simulink model "sampleModel235"  (R2021b)
settings: Solver=VariableStepAuto  StartTime=0.0  StopTime=10.0  RelTol=1e-3
undefined symbols (not defined in the file or in its folder): Newton, Raphson
libraries: simulink x16, slpidlib x3
settings Model: Creator=user  LastModifiedBy=user

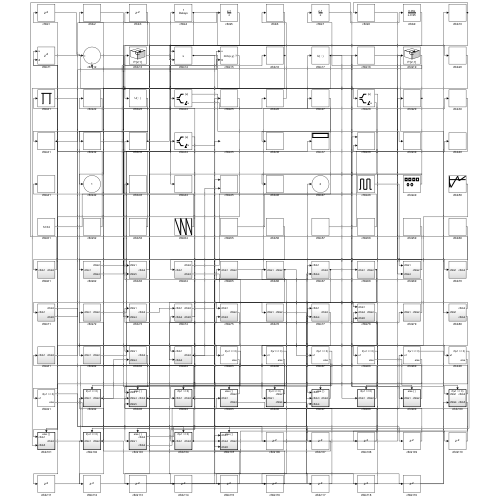
[thumbnail: Simulink's stored preview of the top-level diagram]
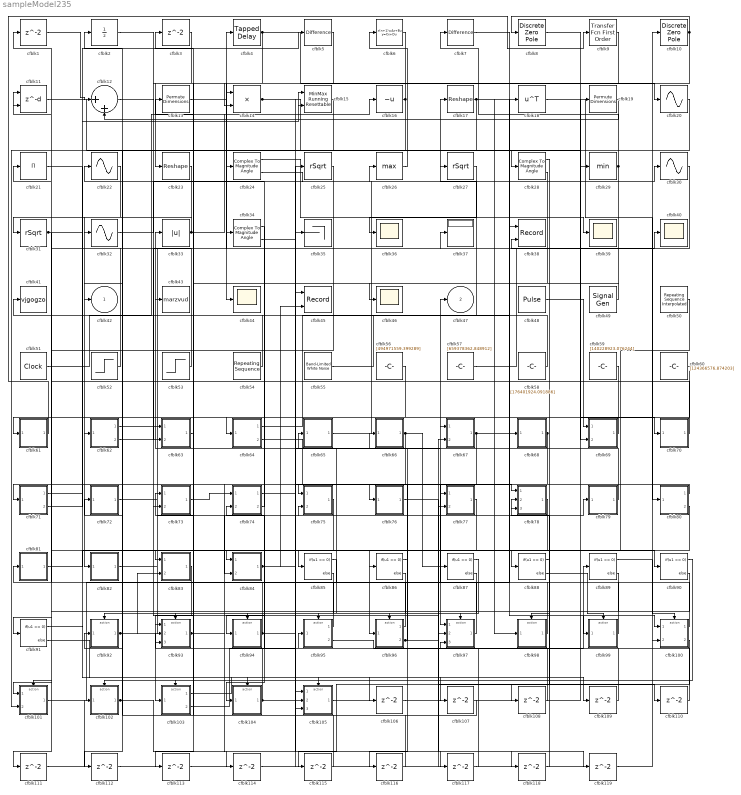
== system sampleModel235 ==
  cfblk{1,3,106..119} (16 alike) : Delay  SampleTime=1
  cfblk10 : DiscreteZeroPole  Poles=[0 0.5]  Gain=1
  cfblk100 : Subsystem  TreatAsAtomicUnit=on
  cfblk101 : Subsystem  TreatAsAtomicUnit=on
  cfblk102 : Subsystem  TreatAsAtomicUnit=on
  cfblk103 : Subsystem  TreatAsAtomicUnit=on
  cfblk104 : Subsystem  TreatAsAtomicUnit=on
  cfblk105 : Subsystem  TreatAsAtomicUnit=on
  cfblk11 : Delay  DelayLengthSource=Input port  SampleTime=1
      settings: InputPortMap=u0,p1
  cfblk12 : Sum  Inputs=|++
  cfblk13 : PermuteDimensions
  cfblk14 : Product
  cfblk15 : simulink/Math Operations/MinMax Running Resettable  Function=min  vinit=0.0
  cfblk16 : UnaryMinus
  cfblk17 : Reshape
  cfblk18 : Math  Operator=transpose  SaturateOnIntegerOverflow=on
  cfblk19 : PermuteDimensions
  cfblk2 : UnitDelay  HasFrameUpgradeWarning=on
  cfblk{20,22,30,32} (4 alike) : Sin  TimeSource=Use external signal  SampleTime=0
  cfblk21 : Product  Inputs=*
  cfblk23 : Reshape
  cfblk24 : ComplexToMagnitudeAngle
  cfblk25 : Sqrt  Operator=rSqrt  AlgorithmType=Newton-Raphson  SaturateOnIntegerOverflow=on
  cfblk26 : MinMax  Function=max
  cfblk27 : Sqrt  Operator=rSqrt  AlgorithmType=Newton-Raphson  SaturateOnIntegerOverflow=on
  cfblk28 : ComplexToMagnitudeAngle
  cfblk29 : MinMax
  cfblk31 : Sqrt  Operator=rSqrt  AlgorithmType=Newton-Raphson  SaturateOnIntegerOverflow=on
  cfblk33 : Abs
  cfblk34 : ComplexToMagnitudeAngle
  cfblk35 : Terminator
  cfblk{36,39..40,44,46} (5 alike) : Scope
  cfblk37 : Display
  cfblk38 : Record  FileSettingsInternal="{\"entries\":[{\"content\":{\"excelSettings\":{\"content\":{},\"type\":\"Streamout.ExcelSettings\"}},\"type\":\"Streamout.FileSettingStorage\",\"uuid\":\"11336398-6d51-4f3b-8d62-29296b9ae9b3\"}],\"packageUris\":[\"http://schema.mathworks.com/mf0/streamout_blocks/R2020a\"],\"version\":\"1.0\"}"  Layout=[1 1]  SignalsInternal="{\"entries\":[{\"content\":{\"signals\":[{\"content\":{\"blockPath\":[\"sampleModel235/cfblk38\"],\"channel\":[],\"dimensions\":[1],\"domain\":\"sampleModel235/cfblk38\",\"lineColor\":\"#a2142f\",\"plots\":[1],\"port\":1,\"sid\":[\"\"],\"signalID\":9263,\"signalName\":\"cfblk101\"},\"type\":\"RecordBlkView.Signal\",\"uuid\":\"63c3850a-55ea-46c7-aea2-e643b16b634b\"},{\"content\":{\"blockPath\":[\"sampleModel235/cfblk38\"],\"channel\":[],\"dimensions\":[1],\"domain\":\"sampleModel235/cfblk38\",\"lineColor\":\"#139fff\",\"plots\":[1],\"port\":2,\"sid\":[\"\"],\"signalID\":9267,\"signalName\":\"cfblk30\"},\"type\":\"RecordBlkView.Signal\",\"uuid\":\"79ddd3dd-8e78-4676-acbe-30bf93b9a830\"}]},\"type\":\"RecordBlkView.InputSignals\",\"uuid\":\"fa292d2c-9bc8-478c-a53f-73bef0c1fc4b\"}],\"packageUris\":[\"http://schema.mathworks.com/mf0/streamout_blocks/R2020a\"],\"version\":\"1.0\"}"  VisualizationBindings="{\"xyplotplugin\":{\"info\":[{\"series\":[{\"bindingParametersList\":[{\"parameter\":\"X-Axis\",\"signalID\":9263,\"signalName\":\"cfblk101\"},{\"parameter\":\"Y-Axis\",\"signalID\":9267,\"signalName\":\"cfblk30\"}],\"seriesID\":30601}],\"subplotID\":1}]}}"  CompatibilityTag=XY
  cfblk4 : simulink/Discrete/Tapped Delay  vinit=0.0  samptime=-1  NumDelays=1  DelayOrder=Oldest  includeCurrent=off
  cfblk41 : ToWorkspace  VariableName=vjgogzo  SaveFormat=Timeseries  SampleTime=-1
  cfblk43 : ToWorkspace  VariableName=marzvud  SaveFormat=Timeseries  SampleTime=-1
  cfblk45 : Record  FileSettingsInternal="{\"entries\":[{\"content\":{\"excelSettings\":{\"content\":{},\"type\":\"Streamout.ExcelSettings\"}},\"type\":\"Streamout.FileSettingStorage\",\"uuid\":\"599320f1-be0e-48c2-8f03-a9a55e95d92d\"}],\"packageUris\":[\"http://schema.mathworks.com/mf0/streamout_blocks/R2020a\"],\"version\":\"1.0\"}"  Layout=[1 1]  SignalsInternal="{\"entries\":[{\"content\":{\"signals\":[{\"content\":{\"blockPath\":[\"sampleModel235/cfblk45\"],\"channel\":[],\"dimensions\":[1],\"domain\":\"sampleModel235/cfblk45\",\"lineColor\":\"#a2142f\",\"plots\":[1],\"port\":1,\"sid\":[\"\"],\"signalID\":9271,\"signalName\":\"cfblk84\"},\"type\":\"RecordBlkView.Signal\",\"uuid\":\"f68cf5d5-64ff-4d75-8381-95ab246270b4\"},{\"content\":{\"blockPath\":[\"sampleModel235/cfblk45\"],\"channel\":[],\"dimensions\":[1],\"domain\":\"sampleModel235/cfblk45\",\"lineColor\":\"#139fff\",\"plots\":[1],\"port\":2,\"sid\":[\"\"],\"signalID\":9275,\"signalName\":\"cfblk84\"},\"type\":\"RecordBlkView.Signal\",\"uuid\":\"4af8da54-8b2c-4738-836e-80062f010a58\"}]},\"type\":\"RecordBlkView.InputSignals\",\"uuid\":\"0d96f0b2-07ca-44bb-ba4c-d588ee9965c7\"}],\"packageUris\":[\"http://schema.mathworks.com/mf0/streamout_blocks/R2020a\"],\"version\":\"1.0\"}"  VisualizationBindings="{\"xyplotplugin\":{\"info\":[{\"series\":[{\"bindingParametersList\":[{\"parameter\":\"X-Axis\",\"signalID\":9271,\"signalName\":\"cfblk84\"},{\"parameter\":\"Y-Axis\",\"signalID\":9275,\"signalName\":\"cfblk84\"}],\"seriesID\":14377}],\"subplotID\":1}]}}"  CompatibilityTag=XY
  cfblk48 : DiscretePulseGenerator  PulseType=Time based  Amplitude=[993990205.841639]  Period=[41434692.825303]  PulseWidth=5  PhaseDelay=[9.000000]
  cfblk49 : SignalGenerator  WaveForm=sawtooth  Amplitude=[-618305415.927345]
  cfblk5 : simulink/Discrete/Difference  ICPrevInput=0.0  OutMin=[]  OutMax=[]  OutDataTypeStr=Inherit: Inherit via back propagation  OutDataType=fixdt(1, 16)  OutScaling=2^-10  DoSatur=off
  cfblk50 : simulink/Sources/Repeating Sequence Interpolated  OutValues=[-355762936.118842, -997864679.690225, 480383751.417807, -129782159.946372, 472491708.446111]  TimeValues=[0 0.1 0.5 0.6 1].'  LookUpMeth=Use Input Below  tsamp=0.01  OutMin=[]  OutMax=[]  OutDataTypeStr=double  OutputDataTypeScalingMode=double  OutDataType=fixdt(0,8)  OutScaling=2^-10
  cfblk51 : DigitalClock
  cfblk52 : Step  Time=[2.000000]  Before=[-898683375.767057]  After=[-744239558.640982]  SampleTime=0
  cfblk53 : Step  Time=[28.000000]  Before=[-372375495.152986]  After=[255511984.528570]  SampleTime=0
  cfblk54 : simulink/Sources/Repeating Sequence  rep_seq_t=[0 2]  rep_seq_y=[659416968.647904, 513787751.748081]
  cfblk55 : simulink/Sources/Band-Limited White Noise  Cov=[2606492098.935749]  Ts=0.1  seed=[8675385123.000000]
  cfblk56 : Constant  Value=[494971559.399289]  SampleTime=1
  cfblk57 : Constant  Value=[659378362.848912]  SampleTime=1
  cfblk58 : Constant  Value=[176401924.091886]  SampleTime=1
  cfblk59 : Constant  Value=[140228923.076244]  SampleTime=1
  cfblk6 : DiscreteStateSpace
  cfblk60 : Constant  Value=[124366576.874203]  SampleTime=1
  cfblk61 : Subsystem
  cfblk62 : Subsystem
  cfblk63 : Subsystem
  cfblk64 : Subsystem
  cfblk65 : Subsystem
  cfblk66 : Subsystem
  cfblk67 : Subsystem
  cfblk68 : Subsystem
  cfblk69 : Subsystem
  cfblk7 : simulink/Discrete/Difference  ICPrevInput=0.0  OutMin=[]  OutMax=[]  OutDataTypeStr=Inherit: Inherit via back propagation  OutDataType=fixdt(1, 16)  OutScaling=2^-10  DoSatur=off
  cfblk70 : Subsystem
  cfblk71 : Subsystem
  cfblk72 : Subsystem
  cfblk73 : Subsystem
  cfblk74 : Subsystem
  cfblk75 : Subsystem
  cfblk76 : Subsystem
  cfblk77 : Subsystem
  cfblk78 : Subsystem
  cfblk79 : Subsystem
  cfblk8 : DiscreteZeroPole  Poles=[0 0.5]  Gain=1
  cfblk80 : Subsystem
  cfblk81 : Subsystem
  cfblk82 : Subsystem
  cfblk83 : Subsystem
  cfblk84 : Subsystem
  cfblk{85..91} (7 alike) : If  IfExpression=u1 >= 0  SampleTime=1
  cfblk9 : simulink/Discrete/Transfer Fcn First Order  PoleZ=0.95  ICPrevOutput=0.0  DoSatur=off
  cfblk92 : Subsystem  TreatAsAtomicUnit=on
  cfblk93 : Subsystem  TreatAsAtomicUnit=on
  cfblk94 : Subsystem  TreatAsAtomicUnit=on
  cfblk95 : Subsystem  TreatAsAtomicUnit=on
  cfblk96 : Subsystem  TreatAsAtomicUnit=on
  cfblk97 : Subsystem  TreatAsAtomicUnit=on
  cfblk98 : Subsystem  TreatAsAtomicUnit=on
  cfblk99 : Subsystem  TreatAsAtomicUnit=on
  cfblk42 : Outport
  cfblk47 : Outport  Port=2
  wires:
  cfblk79/1(cfblk2) -> cfblk33/1
  cfblk51/1 -> cfblk16/1
  cfblk3/1 -> cfblk23/1
  cfblk50/1 -> cfblk88/1
  cfblk22/1 -> cfblk82/1(cfblk1)
  cfblk54/1 -> cfblk41/1
  cfblk10/1 -> cfblk8/1, cfblk14/2
  cfblk101/1(cfblk2) -> cfblk38/1
  cfblk77/1(cfblk2) -> cfblk96/1(cfblk1)
  cfblk13/1 -> cfblk44/1
  cfblk92/1(cfblk2) -> cfblk37/1, cfblk83/2(cfblk4)
  cfblk63/1(cfblk2) -> cfblk13/1
  cfblk73/1(cfblk2) -> cfblk74/1(cfblk1)
  cfblk56/1 -> cfblk64/1(cfblk1)
  cfblk80/1(cfblk2) -> cfblk75/1(cfblk1)
  cfblk82/1(cfblk2) -> cfblk75/2(cfblk3)
  cfblk102/1(cfblk2) -> cfblk72/1(cfblk1), cfblk114/1
  cfblk74/1(cfblk2) -> cfblk76/1(cfblk1)
  cfblk94/1(cfblk2) -> cfblk2/1, cfblk77/1(cfblk1), cfblk106/1
  cfblk55/1 -> cfblk17/1
  cfblk4/1 -> cfblk20/1, cfblk113/1
  cfblk69/1(cfblk2) -> cfblk62/1(cfblk1)
  cfblk33/1 -> cfblk32/1, cfblk15/1
  cfblk83/1(cfblk2) -> cfblk103/1(cfblk1)
  cfblk11/1 -> cfblk28/1
  cfblk30/1 -> cfblk38/2
  cfblk1/1 -> cfblk12/1
  cfblk61/1(cfblk2) -> cfblk9/1
  cfblk72/1(cfblk2) -> cfblk4/1
  cfblk24/1 -> cfblk39/1
  cfblk95/1(cfblk2) -> cfblk21/1
  cfblk15/1 -> cfblk42/1
  cfblk60/1 -> cfblk94/1(cfblk1)
  cfblk9/1 -> cfblk24/1
  cfblk64/1(cfblk2) -> cfblk18/1
  cfblk64/2(cfblk3) -> cfblk78/1(cfblk1)
  cfblk66/1(cfblk2) -> cfblk71/1(cfblk1), cfblk87/1
  cfblk70/1(cfblk2) -> cfblk11/1
  cfblk23/1 -> cfblk31/1
  cfblk65/1(cfblk2) -> cfblk30/1
  cfblk81/1(cfblk2) -> cfblk85/1
  cfblk97/1(cfblk2) -> cfblk47/1
  cfblk27/1 -> cfblk36/1
  cfblk48/1 -> cfblk69/1(cfblk1)
  cfblk8/1 -> cfblk70/1(cfblk1)
  cfblk18/1 -> cfblk80/1(cfblk1)
  cfblk2/1 -> cfblk63/1(cfblk1)
  cfblk52/1 -> cfblk11/2
  cfblk62/1(cfblk2) -> cfblk40/1
  cfblk95/2(cfblk4) -> cfblk89/1
  cfblk5/1 -> cfblk83/1(cfblk1)
  cfblk99/1(cfblk2) -> cfblk78/2(cfblk4)
  cfblk19/1 -> cfblk12/2
  cfblk49/1 -> cfblk46/1
  cfblk31/1 -> cfblk91/1, cfblk15/2
  cfblk80/2(cfblk4) -> cfblk84/1(cfblk1)
  cfblk16/1 -> cfblk14/1, cfblk101/2(cfblk5)
  cfblk67/1(cfblk2) -> cfblk97/1(cfblk1), cfblk99/1(cfblk1)
  cfblk25/1 -> cfblk101/1(cfblk1)
  cfblk71/1(cfblk2) -> cfblk90/1
  cfblk104/1(cfblk2) -> cfblk67/1(cfblk1), cfblk93/2(cfblk4)
  cfblk12/1 -> cfblk97/2(cfblk3)
  cfblk26/1 -> cfblk6/1
  cfblk58/1 -> cfblk43/1
  cfblk103/2(cfblk4) -> cfblk35/1
  cfblk14/1 -> cfblk69/2(cfblk4), cfblk119/1
  cfblk24/2 -> cfblk27/1
  cfblk28/1 -> cfblk61/1(cfblk1)
  cfblk32/1 -> cfblk26/1
  cfblk84/1(cfblk2) -> cfblk45/1, cfblk45/2
  cfblk98/1(cfblk2) -> cfblk66/1(cfblk1)
  cfblk68/1(cfblk2) -> cfblk84/2(cfblk4), cfblk116/1
  cfblk105/1(cfblk2) -> cfblk29/1
  cfblk62/2(cfblk4) -> cfblk34/1
  cfblk57/1 -> cfblk19/1
  cfblk96/1(cfblk2) -> cfblk65/1(cfblk1)
  cfblk78/1(cfblk2) -> cfblk86/1
  cfblk29/1 -> cfblk7/1, cfblk108/1
  cfblk53/1 -> cfblk1/1
  cfblk6/1 -> cfblk63/2(cfblk5)
  cfblk34/1 -> cfblk104/1(cfblk1)
  cfblk93/1(cfblk2) -> cfblk79/1(cfblk1), cfblk117/1
  cfblk96/2(cfblk4) -> cfblk81/1(cfblk1), cfblk118/1
  cfblk34/2 -> cfblk25/1
  cfblk100/1(cfblk2) -> cfblk73/1(cfblk1)
  cfblk7/1 -> cfblk68/1(cfblk1)
  cfblk59/1 -> cfblk105/3(cfblk5)
  cfblk74/2(cfblk5) -> cfblk22/1
  cfblk71/2(cfblk5) -> cfblk5/1
  cfblk28/2 -> cfblk93/1(cfblk1)
  cfblk17/1 -> cfblk73/2(cfblk4), cfblk98/1(cfblk1), cfblk100/1(cfblk1)
  cfblk85/1 -> cfblk92/Action
  cfblk85/2 -> cfblk93/Action
  cfblk86/1 -> cfblk94/Action
  cfblk86/2 -> cfblk95/Action
  cfblk87/1 -> cfblk96/Action
  cfblk87/2 -> cfblk97/Action
  cfblk88/1 -> cfblk98/Action
  cfblk88/2 -> cfblk99/Action
  cfblk89/1 -> cfblk100/Action
  cfblk89/2 -> cfblk101/Action
  cfblk90/1 -> cfblk102/Action
  cfblk90/2 -> cfblk103/Action
  cfblk91/1 -> cfblk104/Action
  cfblk91/2 -> cfblk105/Action
  cfblk106/1 -> cfblk67/2(cfblk4)
  cfblk103/1(cfblk2) -> cfblk107/1
  cfblk107/1 -> cfblk105/2(cfblk4)
  cfblk108/1 -> cfblk95/1(cfblk1)
  cfblk21/1 -> cfblk109/1
  cfblk109/1 -> cfblk3/1
  cfblk76/1(cfblk2) -> cfblk110/1
  cfblk110/1 -> cfblk74/2(cfblk4)
  cfblk75/1(cfblk2) -> cfblk111/1
  cfblk111/1 -> cfblk102/1(cfblk1)
  cfblk20/1 -> cfblk112/1
  cfblk112/1 -> cfblk105/1(cfblk1)
  cfblk113/1 -> cfblk100/2(cfblk4)
  cfblk114/1 -> cfblk77/2(cfblk4)
  cfblk100/2(cfblk5) -> cfblk115/1
  cfblk115/1 -> cfblk92/1(cfblk1)
  cfblk116/1 -> cfblk93/3(cfblk5)
  cfblk117/1 -> cfblk97/3(cfblk4)
  cfblk118/1 -> cfblk78/3(cfblk5)
  cfblk119/1 -> cfblk10/1

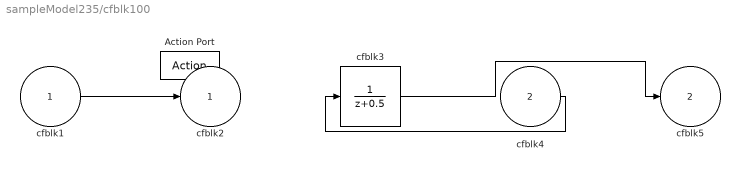
== system sampleModel235/cfblk100 ==
  cfblk1 : Inport
  cfblk4 : Inport  Port=2
  Action Port : ActionPort  ActionPortLabel=if(u1 >= 0)
  cfblk3 : DiscreteTransferFcn
  cfblk2 : Outport
  cfblk5 : Outport  Port=2
  wires:
  cfblk1/1 -> cfblk2/1
  cfblk3/1 -> cfblk5/1
  cfblk4/1 -> cfblk3/1

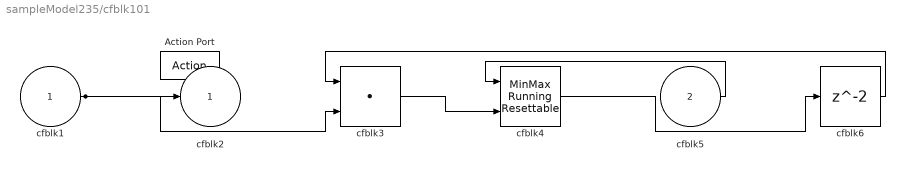
== system sampleModel235/cfblk101 ==
  cfblk1 : Inport
  cfblk5 : Inport  Port=2
  Action Port : ActionPort  ActionPortLabel=else
  cfblk3 : DotProduct  InputSameDT=on  OutDataTypeStr=Inherit: Inherit via internal rule
  cfblk4 : simulink/Math Operations/MinMax Running Resettable  Function=min  vinit=0.0
  cfblk6 : Delay
  cfblk2 : Outport
  wires:
  cfblk5/1 -> cfblk4/1
  cfblk3/1 -> cfblk4/2
  cfblk1/1 -> cfblk2/1, cfblk3/2
  cfblk4/1 -> cfblk6/1
  cfblk6/1 -> cfblk3/1

== system sampleModel235/cfblk102 ==
  cfblk1 : Inport
  Action Port : ActionPort  ActionPortLabel=if(u1 >= 0)
  cfblk3 : Constant  Value=[-162159908.679487]  SampleTime=1
  cfblk2 : Outport
  wires:
  cfblk1/1 -> cfblk2/1

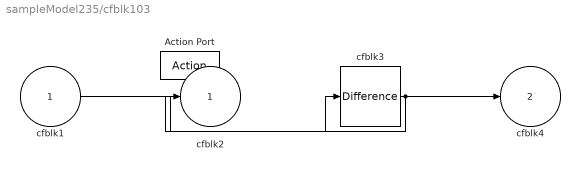
== system sampleModel235/cfblk103 ==
  cfblk1 : Inport
  Action Port : ActionPort  ActionPortLabel=else
  cfblk3 : simulink/Discrete/Difference  ICPrevInput=0.0  OutMin=[]  OutMax=[]  OutDataTypeStr=Inherit: Inherit via back propagation  OutDataType=fixdt(1, 16)  OutScaling=2^-10  DoSatur=off
  cfblk2 : Outport
  cfblk4 : Outport  Port=2
  wires:
  cfblk1/1 -> cfblk3/1
  cfblk3/1 -> cfblk4/1, cfblk2/1

== system sampleModel235/cfblk104 ==
  cfblk1 : Inport
  Action Port : ActionPort  ActionPortLabel=if(u1 >= 0)
  cfblk3 : Sin  TimeSource=Use external signal  SampleTime=0
  cfblk2 : Outport
  wires:
  cfblk3/1 -> cfblk2/1
  cfblk1/1 -> cfblk3/1

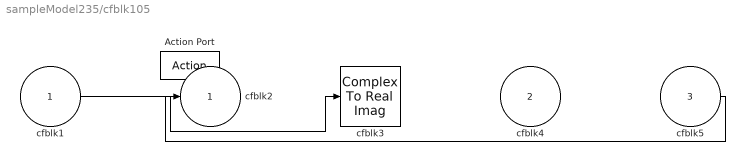
== system sampleModel235/cfblk105 ==
  cfblk1 : Inport
  cfblk4 : Inport  Port=2
  cfblk5 : Inport  Port=3
  Action Port : ActionPort  ActionPortLabel=else
  cfblk3 : ComplexToRealImag
  cfblk2 : Outport
  wires:
  cfblk1/1 -> cfblk3/1
  cfblk5/1 -> cfblk2/1

== system sampleModel235/cfblk61 ==
  cfblk1 : Inport
  cfblk3 : Bias  Bias=[-453538198.164832]
  cfblk2 : Outport
  wires:
  cfblk1/1 -> cfblk3/1
  cfblk3/1 -> cfblk2/1

== system sampleModel235/cfblk62 ==
  cfblk1 : Inport
  cfblk3 : Sum  Inputs=|++
  cfblk2 : Outport
  cfblk4 : Outport  Port=2
  wires:
  cfblk3/1 -> cfblk4/1, cfblk2/1
  cfblk1/1 -> cfblk3/1, cfblk3/2

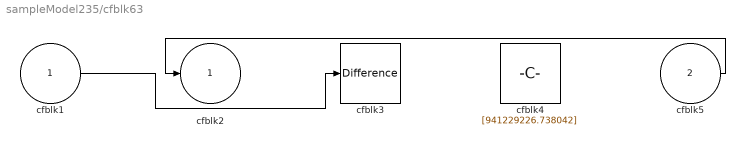
== system sampleModel235/cfblk63 ==
  cfblk1 : Inport
  cfblk5 : Inport  Port=2
  cfblk3 : simulink/Discrete/Difference  ICPrevInput=0.0  OutMin=[]  OutMax=[]  OutDataTypeStr=Inherit: Inherit via back propagation  OutDataType=fixdt(1, 16)  OutScaling=2^-10  DoSatur=off
  cfblk4 : Constant  Value=[941229226.738042]  SampleTime=1
  cfblk2 : Outport
  wires:
  cfblk5/1 -> cfblk2/1
  cfblk1/1 -> cfblk3/1

== system sampleModel235/cfblk64 ==
  cfblk1 : Inport
  cfblk2 : Outport
  cfblk3 : Outport  Port=2
  wires:
  cfblk1/1 -> cfblk2/1, cfblk3/1

== system sampleModel235/cfblk65 ==
  cfblk1 : Inport
  cfblk3 : Delay  DelayLengthSource=Input port  SampleTime=1
      settings: InputPortMap=u0,p1
  cfblk4 : simulink/Math Operations/Slider Gain  gain=1  low=0  high=2
  cfblk2 : Outport
  wires:
  cfblk1/1 -> cfblk4/1, cfblk3/2
  cfblk4/1 -> cfblk3/1
  cfblk3/1 -> cfblk2/1

== system sampleModel235/cfblk66 ==
  cfblk1 : Inport
  cfblk3 : slpidlib/PID Controller  Controller=PID  Form=Parallel  TimeDomain=Discrete-time  UseExternalTs=off  SampleTime=1  IntegratorMethod=Forward Euler  FilterMethod=Forward Euler  ControllerParametersSource=internal  P=1  I=1  D=0  UseFilter=on  N=100  TunerSelectOption=Transfer Function Based (PID Tuner App)  InitialConditionSource=internal  InitialConditionForIntegrator=0  InitialConditionForFilter=0  DifferentiatorICPrevScaledInput=0  ExternalReset=none  TrackingMode=off  Kt=1  LimitOutput=off  SatLimitsSource=internal  UpperSaturationLimit=inf  LowerSaturationLimit=-inf  LinearizeAsGain=off  AntiWindupMode=none  Kb=1  POutMin=[]  POutMax=[]  IOutMin=[]  IOutMax=[]  DOutMin=[]  DOutMax=[]  NOutMin=[]  NOutMax=[]  SumOutMin=[]  SumOutMax=[]  SaturationOutMin=[]  SaturationOutMax=[]  PParamMin=[]  PParamMax=[]  IParamMin=[]  IParamMax=[]  DParamMin=[]  DParamMax=[]  NParamMin=[]  NParamMax=[]  KbParamMin=[]  KbParamMax=[]  KtParamMin=[]  KtParamMax=[]  KbOutMin=[]  KbOutMax=[]  KtOutMin=[]  KtOutMax=[]  IntegratorOutMin=[]  IntegratorOutMax=[]  FilterOutMin=[]  FilterOutMax=[]  SumI1OutMin=[]  SumI1OutMax=[]  SumI2OutMin=[]  SumI2OutMax=[]  SumI3OutMin=[]  SumI3OutMax=[]  SumI4OutMin=[]  SumI4OutMax=[]  SumDOutMin=[]  SumDOutMax=[]  DifferentiatorOutMin=[]  DifferentiatorOutMax=[]  FilterDiffOutCoefMin=[]  FilterDiffOutCoefMax=[]  ReciprocalOutMin=[]  ReciprocalOutMax=[]  SumDenOutMin=[]  SumDenOutMax=[]  SumNumOutMin=[]  SumNumOutMax=[]  DivideOutMin=[]  DivideOutMax=[]  UdiffTsProdOutMin=[]  UdiffTsProdOutMax=[]  NTsProdOutMin=[]  NTsProdOutMax=[]  UintegralTsProdOutMin=[]  UintegralTsProdOutMax=[]  UngainTsProdOutMin=[]  UngainTsProdOutMax=[]  IntegratorContinuousStateAttributes=''  IntegratorStateMustResolveToSignalObject=off  IntegratorRTWStateStorageClass=Auto  FilterContinuousStateAttributes=''  FilterStateMustResolveToSignalObject=off  FilterRTWStateStorageClass=Auto  ParallelPVariant=InternalParameters  IdealPVariant=Disabled  IVariant=InternalParameters  DVariant=InternalParameters  IntegratorVariant=Discrete  SatVariant=Disabled  AWVariant=Passthrough  PCopyVariant=Disabled  TRVariant=Disabled  FdbkBlocksVariant=Forward  IdealPFdbkVariant=Disabled  SatFdbkVariant=Disabled  DerivativeFilterVariant=ForwardEulerFilter  NVariant=InternalParameters  NCopyVariant=Disabled  FilterICVariant=InternalICsFilter  IntegratorICVariant=InternalICs  ExternalResetVariant=Disabled  TRSumVariant=Passthrough  SumFdbkVariant=Disabled  SumVariant=Sum_PID  TsampFilterVariant=InternalTs  TsampNgainVariant=Passthrough  TsampIntegralVariant=Passthrough  ExternalSaturationOutDataTypeStr=Inherit: Same as second input
  cfblk4 : Gain  Gain=[432391618.383563]
  cfblk2 : Outport
  wires:
  cfblk3/1 -> cfblk4/1
  cfblk4/1 -> cfblk2/1
  cfblk1/1 -> cfblk3/1

== system sampleModel235/cfblk67 ==
  cfblk1 : Inport
  cfblk4 : Inport  Port=2
  cfblk3 : Sqrt  SaturateOnIntegerOverflow=on
  cfblk2 : Outport
  wires:
  cfblk3/1 -> cfblk2/1
  cfblk1/1 -> cfblk3/1

== system sampleModel235/cfblk68 ==
  cfblk1 : Inport
  cfblk3 : ComplexToRealImag
  cfblk2 : Outport
  wires:
  cfblk1/1 -> cfblk3/1
  cfblk3/1 -> cfblk2/1

== system sampleModel235/cfblk69 ==
  cfblk1 : Inport
  cfblk4 : Inport  Port=2
  cfblk3 : MinMax  Inputs=2
  cfblk2 : Outport
  wires:
  cfblk4/1 -> cfblk3/1
  cfblk1/1 -> cfblk3/2
  cfblk3/1 -> cfblk2/1

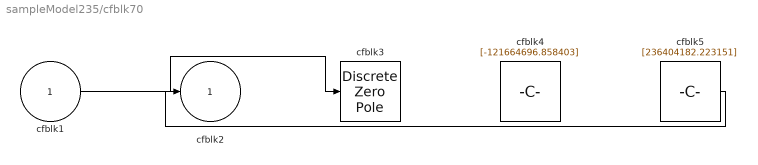
== system sampleModel235/cfblk70 ==
  cfblk1 : Inport
  cfblk3 : DiscreteZeroPole  Poles=[0 0.5]  Gain=1
  cfblk4 : Constant  Value=[-121664696.858403]  SampleTime=1
  cfblk5 : Constant  Value=[236404182.223151]  SampleTime=1
  cfblk2 : Outport
  wires:
  cfblk1/1 -> cfblk3/1
  cfblk5/1 -> cfblk2/1

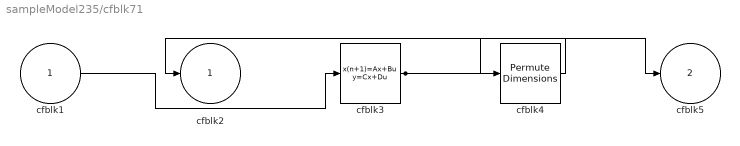
== system sampleModel235/cfblk71 ==
  cfblk1 : Inport
  cfblk3 : DiscreteStateSpace
  cfblk4 : PermuteDimensions
  cfblk2 : Outport
  cfblk5 : Outport  Port=2
  wires:
  cfblk3/1 -> cfblk4/1, cfblk5/1
  cfblk4/1 -> cfblk2/1
  cfblk1/1 -> cfblk3/1

== system sampleModel235/cfblk72 ==
  cfblk1 : Inport
  cfblk3 : Gain  Gain=[948862798.807821]
  cfblk2 : Outport
  wires:
  cfblk3/1 -> cfblk2/1
  cfblk1/1 -> cfblk3/1

== system sampleModel235/cfblk73 ==
  cfblk1 : Inport
  cfblk4 : Inport  Port=2
  cfblk3 : UnitDelay  HasFrameUpgradeWarning=on
  cfblk2 : Outport
  wires:
  cfblk4/1 -> cfblk3/1
  cfblk3/1 -> cfblk2/1

== system sampleModel235/cfblk74 ==
  cfblk1 : Inport
  cfblk4 : Inport  Port=2
  cfblk3 : DiscreteFilter  SampleTime=1
  cfblk2 : Outport
  cfblk5 : Outport  Port=2
  wires:
  cfblk1/1 -> cfblk3/1
  cfblk4/1 -> cfblk5/1
  cfblk3/1 -> cfblk2/1

== system sampleModel235/cfblk75 ==
  cfblk1 : Inport
  cfblk3 : Inport  Port=2
  cfblk2 : Outport
  wires:
  cfblk1/1 -> cfblk2/1

== system sampleModel235/cfblk76 ==
  cfblk1 : Inport
  cfblk3 : simulink/Discrete/Transfer Fcn Real Zero  ZeroZ=0.75  ICPrevInput=0.0  DoSatur=off
      settings: SourceProductBaseCode=SL
  cfblk4 : Delay  ShowEnablePort=on  SampleTime=1
      settings: InputPortMap=u0,e6
  cfblk5 : Constant  Value=[-99394838.353341]  SampleTime=1
  cfblk2 : Outport
  wires:
  cfblk1/1 -> cfblk3/1
  cfblk3/1 -> cfblk2/1
  cfblk5/1 -> cfblk4/1, cfblk4/2

== system sampleModel235/cfblk77 ==
  cfblk1 : Inport
  cfblk4 : Inport  Port=2
  cfblk3 : Constant  Value=[766673496.063240]  SampleTime=1
  cfblk2 : Outport
  wires:
  cfblk3/1 -> cfblk2/1

== system sampleModel235/cfblk78 ==
  cfblk1 : Inport
  cfblk4 : Inport  Port=2
  cfblk5 : Inport  Port=3
  cfblk3 : Constant  Value=[-757795935.160757]  SampleTime=1
  cfblk2 : Outport
  wires:
  cfblk4/1 -> cfblk2/1

== system sampleModel235/cfblk79 ==
  cfblk1 : Inport
  cfblk3 : DotProduct  InputSameDT=on  OutDataTypeStr=Inherit: Inherit via internal rule
  cfblk2 : Outport
  wires:
  cfblk1/1 -> cfblk3/1, cfblk3/2
  cfblk3/1 -> cfblk2/1

== system sampleModel235/cfblk80 ==
  cfblk1 : Inport
  cfblk3 : Assignment  DiagnosticForDimensions=Warning  IndexOptions=Index vector (dialog)  Indices=1  OutputSizes=1
  cfblk2 : Outport
  cfblk4 : Outport  Port=2
  wires:
  cfblk1/1 -> cfblk4/1, cfblk3/1, cfblk3/2
  cfblk3/1 -> cfblk2/1

== system sampleModel235/cfblk81 ==
  cfblk1 : Inport
  cfblk3 : DiscreteFir  SampleTime=1
  cfblk2 : Outport
  wires:
  cfblk1/1 -> cfblk3/1
  cfblk3/1 -> cfblk2/1

== system sampleModel235/cfblk82 ==
  cfblk1 : Inport
  cfblk3 : DiscreteTransferFcn  SampleTime=1
  cfblk4 : slpidlib/PID Controller  Controller=PID  Form=Parallel  TimeDomain=Discrete-time  UseExternalTs=off  SampleTime=1  IntegratorMethod=Forward Euler  FilterMethod=Forward Euler  ControllerParametersSource=internal  P=1  I=1  D=0  UseFilter=on  N=100  TunerSelectOption=Transfer Function Based (PID Tuner App)  InitialConditionSource=internal  InitialConditionForIntegrator=0  InitialConditionForFilter=0  DifferentiatorICPrevScaledInput=0  ExternalReset=none  TrackingMode=off  Kt=1  LimitOutput=off  SatLimitsSource=internal  UpperSaturationLimit=inf  LowerSaturationLimit=-inf  LinearizeAsGain=off  AntiWindupMode=none  Kb=1  POutMin=[]  POutMax=[]  IOutMin=[]  IOutMax=[]  DOutMin=[]  DOutMax=[]  NOutMin=[]  NOutMax=[]  SumOutMin=[]  SumOutMax=[]  SaturationOutMin=[]  SaturationOutMax=[]  PParamMin=[]  PParamMax=[]  IParamMin=[]  IParamMax=[]  DParamMin=[]  DParamMax=[]  NParamMin=[]  NParamMax=[]  KbParamMin=[]  KbParamMax=[]  KtParamMin=[]  KtParamMax=[]  KbOutMin=[]  KbOutMax=[]  KtOutMin=[]  KtOutMax=[]  IntegratorOutMin=[]  IntegratorOutMax=[]  FilterOutMin=[]  FilterOutMax=[]  SumI1OutMin=[]  SumI1OutMax=[]  SumI2OutMin=[]  SumI2OutMax=[]  SumI3OutMin=[]  SumI3OutMax=[]  SumI4OutMin=[]  SumI4OutMax=[]  SumDOutMin=[]  SumDOutMax=[]  DifferentiatorOutMin=[]  DifferentiatorOutMax=[]  FilterDiffOutCoefMin=[]  FilterDiffOutCoefMax=[]  ReciprocalOutMin=[]  ReciprocalOutMax=[]  SumDenOutMin=[]  SumDenOutMax=[]  SumNumOutMin=[]  SumNumOutMax=[]  DivideOutMin=[]  DivideOutMax=[]  UdiffTsProdOutMin=[]  UdiffTsProdOutMax=[]  NTsProdOutMin=[]  NTsProdOutMax=[]  UintegralTsProdOutMin=[]  UintegralTsProdOutMax=[]  UngainTsProdOutMin=[]  UngainTsProdOutMax=[]  IntegratorContinuousStateAttributes=''  IntegratorStateMustResolveToSignalObject=off  IntegratorRTWStateStorageClass=Auto  FilterContinuousStateAttributes=''  FilterStateMustResolveToSignalObject=off  FilterRTWStateStorageClass=Auto  ParallelPVariant=InternalParameters  IdealPVariant=Disabled  IVariant=InternalParameters  DVariant=InternalParameters  IntegratorVariant=Discrete  SatVariant=Disabled  AWVariant=Passthrough  PCopyVariant=Disabled  TRVariant=Disabled  FdbkBlocksVariant=Forward  IdealPFdbkVariant=Disabled  SatFdbkVariant=Disabled  DerivativeFilterVariant=ForwardEulerFilter  NVariant=InternalParameters  NCopyVariant=Disabled  FilterICVariant=InternalICsFilter  IntegratorICVariant=InternalICs  ExternalResetVariant=Disabled  TRSumVariant=Passthrough  SumFdbkVariant=Disabled  SumVariant=Sum_PID  TsampFilterVariant=InternalTs  TsampNgainVariant=Passthrough  TsampIntegralVariant=Passthrough  ExternalSaturationOutDataTypeStr=Inherit: Same as second input
  cfblk2 : Outport
  wires:
  cfblk1/1 -> cfblk4/1
  cfblk4/1 -> cfblk3/1
  cfblk3/1 -> cfblk2/1

== system sampleModel235/cfblk83 ==
  cfblk1 : Inport
  cfblk4 : Inport  Port=2
  cfblk3 : Polyval  Coefs=[ +2.081618890e-019, -1.441693666e-014, +4.719686976e-010, -8.536869453e-006, +1.621573104e-001, -8.087801117e+001 ]
  cfblk2 : Outport
  wires:
  cfblk4/1 -> cfblk3/1
  cfblk1/1 -> cfblk2/1

== system sampleModel235/cfblk84 ==
  cfblk1 : Inport
  cfblk4 : Inport  Port=2
  cfblk3 : ComplexToRealImag
  cfblk2 : Outport
  wires:
  cfblk1/1 -> cfblk3/1
  cfblk4/1 -> cfblk2/1

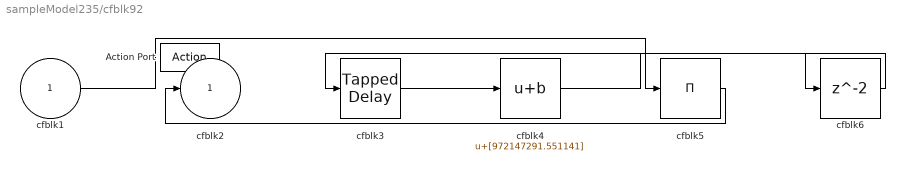
== system sampleModel235/cfblk92 ==
  cfblk1 : Inport
  Action Port : ActionPort  ActionPortLabel=if(u1 >= 0)
  cfblk3 : simulink/Discrete/Tapped Delay  vinit=0.0  samptime=-1  NumDelays=1  DelayOrder=Oldest  includeCurrent=off
  cfblk4 : Bias  Bias=[972147291.551141]
  cfblk5 : Product  Inputs=*
  cfblk6 : Delay
  cfblk2 : Outport
  wires:
  cfblk3/1 -> cfblk4/1
  cfblk5/1 -> cfblk2/1
  cfblk1/1 -> cfblk5/1
  cfblk4/1 -> cfblk6/1
  cfblk6/1 -> cfblk3/1

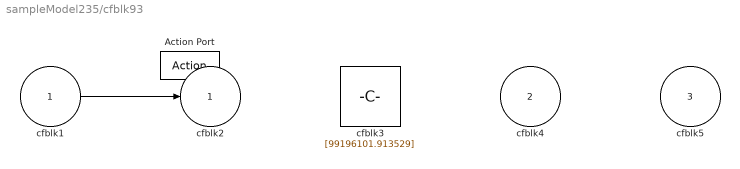
== system sampleModel235/cfblk93 ==
  cfblk1 : Inport
  cfblk4 : Inport  Port=2
  cfblk5 : Inport  Port=3
  Action Port : ActionPort  ActionPortLabel=else
  cfblk3 : Constant  Value=[99196101.913529]  SampleTime=1
  cfblk2 : Outport
  wires:
  cfblk1/1 -> cfblk2/1

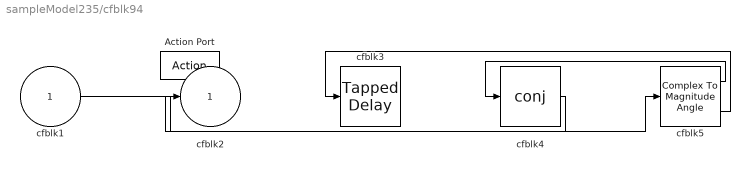
== system sampleModel235/cfblk94 ==
  cfblk1 : Inport
  Action Port : ActionPort  ActionPortLabel=if(u1 >= 0)
  cfblk3 : simulink/Discrete/Tapped Delay  vinit=0.0  samptime=-1  NumDelays=1  DelayOrder=Oldest  includeCurrent=off
  cfblk4 : Math  Operator=conj  SaturateOnIntegerOverflow=on
  cfblk5 : ComplexToMagnitudeAngle
  cfblk2 : Outport
  wires:
  cfblk5/1 -> cfblk4/1
  cfblk1/1 -> cfblk5/1
  cfblk5/2 -> cfblk3/1
  cfblk4/1 -> cfblk2/1

== system sampleModel235/cfblk95 ==
  cfblk1 : Inport
  Action Port : ActionPort  ActionPortLabel=else
  cfblk3 : Signum
  cfblk2 : Outport
  cfblk4 : Outport  Port=2
  wires:
  cfblk1/1 -> cfblk4/1, cfblk3/1
  cfblk3/1 -> cfblk2/1

== system sampleModel235/cfblk96 ==
  cfblk1 : Inport
  Action Port : ActionPort  ActionPortLabel=if(u1 >= 0)
  cfblk3 : Constant  Value=[-348433426.404080]  SampleTime=1
  cfblk2 : Outport
  cfblk4 : Outport  Port=2
  wires:
  cfblk1/1 -> cfblk2/1
  cfblk3/1 -> cfblk4/1

== system sampleModel235/cfblk97 ==
  cfblk1 : Inport
  cfblk3 : Inport  Port=2
  cfblk4 : Inport  Port=3
  Action Port : ActionPort  ActionPortLabel=else
  cfblk2 : Outport
  wires:
  cfblk1/1 -> cfblk2/1

== system sampleModel235/cfblk98 ==
  cfblk1 : Inport
  Action Port : ActionPort  ActionPortLabel=if(u1 >= 0)
  cfblk3 : slpidlib/PID Controller (2DOF)  Controller=PID  Form=Parallel  TimeDomain=Discrete-time  UseExternalTs=off  SampleTime=-1  IntegratorMethod=Forward Euler  FilterMethod=Forward Euler  ControllerParametersSource=internal  P=1  I=1  D=0  UseFilter=on  N=100  b=1  c=1  TunerSelectOption=Transfer Function Based (PID Tuner App)  InitialConditionSource=internal  InitialConditionForIntegrator=0  InitialConditionForFilter=0  DifferentiatorICPrevScaledInput=0  ExternalReset=none  TrackingMode=off  Kt=1  LimitOutput=off  SatLimitsSource=internal  UpperSaturationLimit=inf  LowerSaturationLimit=-inf  LinearizeAsGain=off  AntiWindupMode=none  Kb=1  POutMin=[]  POutMax=[]  IOutMin=[]  IOutMax=[]  DOutMin=[]  DOutMax=[]  NOutMin=[]  NOutMax=[]  bOutMin=[]  bOutMax=[]  cOutMin=[]  cOutMax=[]  SumOutMin=[]  SumOutMax=[]  SaturationOutMin=[]  SaturationOutMax=[]  PParamMin=[]  PParamMax=[]  IParamMin=[]  IParamMax=[]  DParamMin=[]  DParamMax=[]  NParamMin=[]  NParamMax=[]  bParamMin=[]  bParamMax=[]  cParamMin=[]  cParamMax=[]  KbParamMin=[]  KbParamMax=[]  KtParamMin=[]  KtParamMax=[]  KbOutMin=[]  KbOutMax=[]  KtOutMin=[]  KtOutMax=[]  IntegratorOutMin=[]  IntegratorOutMax=[]  FilterOutMin=[]  FilterOutMax=[]  SumI1OutMin=[]  SumI1OutMax=[]  SumI2OutMin=[]  SumI2OutMax=[]  SumI3OutMin=[]  SumI3OutMax=[]  SumI4OutMin=[]  SumI4OutMax=[]  SumDOutMin=[]  SumDOutMax=[]  Sum1OutMin=[]  Sum1OutMax=[]  Sum2OutMin=[]  Sum2OutMax=[]  Sum3OutMin=[]  Sum3OutMax=[]  DifferentiatorOutMin=[]  DifferentiatorOutMax=[]  FilterDiffOutCoefMin=[]  FilterDiffOutCoefMax=[]  ReciprocalOutMin=[]  ReciprocalOutMax=[]  SumDenOutMin=[]  SumDenOutMax=[]  SumNumOutMin=[]  SumNumOutMax=[]  DivideOutMin=[]  DivideOutMax=[]  UdiffTsProdOutMin=[]  UdiffTsProdOutMax=[]  NTsProdOutMin=[]  NTsProdOutMax=[]  UintegralTsProdOutMin=[]  UintegralTsProdOutMax=[]  UngainTsProdOutMin=[]  UngainTsProdOutMax=[]  IntegratorContinuousStateAttributes=''  IntegratorStateMustResolveToSignalObject=off  IntegratorRTWStateStorageClass=Auto  FilterContinuousStateAttributes=''  FilterStateMustResolveToSignalObject=off  FilterRTWStateStorageClass=Auto  ParallelPVariant=InternalParameters  IdealPVariant=Disabled  IVariant=InternalParameters  DVariant=InternalParameters  bVariant=InternalParameters  cVariant=InternalParameters  IntegratorVariant=Discrete  SatVariant=Disabled  AWVariant=Passthrough  PCopyVariant=Disabled  TRVariant=Disabled  FdbkBlocksVariant=Forward  IdealPFdbkVariant=Disabled  SatFdbkVariant=Disabled  DerivativeFilterVariant=ForwardEulerFilter  NVariant=InternalParameters  NCopyVariant=Disabled  FilterICVariant=InternalICsFilter  IntegratorICVariant=InternalICs  ExternalResetVariant=Disabled  TRSumVariant=Passthrough  SumFdbkVariant=Disabled  SumVariant=Sum_PID  TsampFilterVariant=InternalTs  TsampNgainVariant=Passthrough  TsampIntegralVariant=Passthrough  ExternalSaturationOutDataTypeStr=Inherit: Same as second input
      settings: SourceProductBaseCode=SL
  cfblk4 : Bias  Bias=[-92562294.972788]
  cfblk2 : Outport
  wires:
  cfblk4/1 -> cfblk3/1
  cfblk1/1 -> cfblk4/1, cfblk3/2
  cfblk3/1 -> cfblk2/1

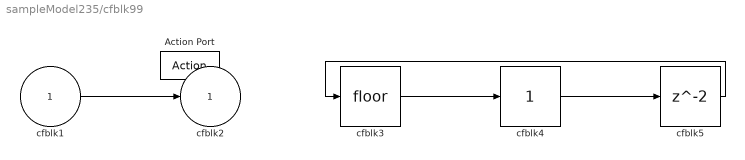
== system sampleModel235/cfblk99 ==
  cfblk1 : Inport
  Action Port : ActionPort  ActionPortLabel=else
  cfblk3 : Rounding
  cfblk4 : simulink/Math Operations/Slider Gain  gain=1  low=0  high=2
  cfblk5 : Delay
  cfblk2 : Outport
  wires:
  cfblk1/1 -> cfblk2/1
  cfblk3/1 -> cfblk4/1
  cfblk4/1 -> cfblk5/1
  cfblk5/1 -> cfblk3/1
